simulink model "R_soft_sim2020b"  (R2021a)
settings: Solver=VariableStepAuto  StartTime=0.0  StopTime=10  FixedStep=0.0001  RelTol=1e-3
values from neighbouring files (symbols this model uses):
  beta = 0.1    [computational_time.m]    (also in final_simulation.m; init_script.m)
  beta_r = 0.5    [final_simulation.m]
  D = 0.1    [computational_time.m]    (also in dampingMatrix.m = reshape([0.0,0.0,0.0,0.0,beta,t2,0.0,t2,beta./3.0],[3,3]); final_simulation.m; init_script.m; multiple_frame_plot.m)
  g = 9.81    [computational_time.m]    (also in final_simulation.m; init_script.m)
  k = 1    [computational_time.m]    (also in final_simulation.m; init_script.m = 0.1)
  Kd = -K(2)    [final_simulation.m]
  Kp = -K(1)    [final_simulation.m]
  L = 1    [computational_time.m]    (also in coriolisMatrix.m = ct{1}; final_simulation.m; init_script.m; multiple_frame_plot.m)
  m = 1    [computational_time.m]    (also in coriolisMatrix.m = ct{2}; final_simulation.m; init_script.m)
  theta_dot_init = zeros(3, 1)    [final_simulation.m]
  theta_init = [0; pi/4; -pi/4]    [final_simulation.m]
undefined symbols (not defined in the file or in its folder): alpha_des, collocatedFL, collocatedFL2, DiscIntNeverNeededParam, RSoft_dynamics, Soft_dynamics, thetaR_des
libraries: spsTriangleGeneratorLib x1
settings Model: Creator=Utente  LastModifiedBy=Utente

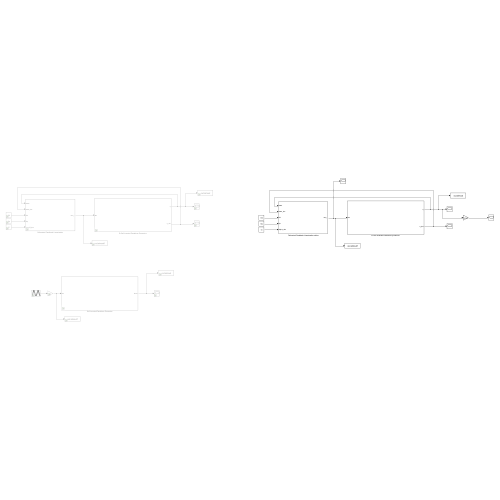
[thumbnail: Simulink's stored preview of the top-level diagram]
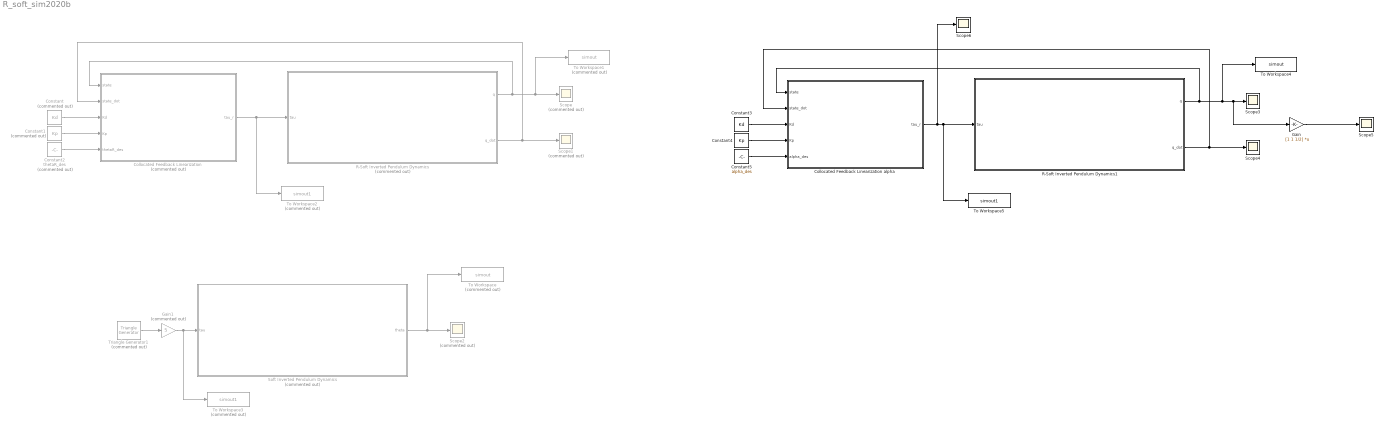
== system R_soft_sim2020b ==
  Collocated Feedback Linearization : Subsystem  Commented=on
  Collocated Feedback Linearization alpha : Subsystem
  Constant : Constant  Commented=on  Value=Kd
  Constant1 : Constant  Commented=on  Value=Kp
  Constant2 : Constant  Commented=on  Value=thetaR_des
  Constant3 : Constant  Value=Kd
  Constant4 : Constant  Value=Kp
  Constant5 : Constant  Value=alpha_des
  Gain : Gain  Gain=[1 1 1/2]  Multiplication=Matrix(K*u) (u vector)
  Gain1 : Gain  Commented=on  Gain=5
  R-Soft Inverted Pendulum Dynamics : Subsystem  Commented=on
  R-Soft Inverted Pendulum Dynamics1 : Subsystem
  Scope : Scope  Commented=on
  Scope1 : Scope  Commented=on
  Scope2 : Scope  Commented=on
  Scope{3..6} (4 alike) : Scope
  Soft Inverted Pendulum Dynamics : Subsystem  Commented=on
  To Workspace : ToWorkspace  Commented=on  VariableName=simout  SaveFormat=Timeseries  SampleTime=-1
  To Workspace1 : ToWorkspace  Commented=on  VariableName=simout  SaveFormat=Timeseries  SampleTime=-1
  To Workspace2 : ToWorkspace  Commented=on  VariableName=simout1  SaveFormat=Timeseries  SampleTime=-1
  To Workspace3 : ToWorkspace  Commented=on  VariableName=simout1  SaveFormat=Timeseries  SampleTime=-1
  To Workspace4 : ToWorkspace  VariableName=simout  SaveFormat=Timeseries  SampleTime=-1
  To Workspace5 : ToWorkspace  VariableName=simout1  SaveFormat=Timeseries  SampleTime=-1
  Triangle Generator1 : spsTriangleGeneratorLib/Triangle Generator  Commented=on  Freq=1/180  Phase=0  Ts=0
  wires:
  Gain1/1 -> To Workspace3/1, Soft Inverted Pendulum Dynamics/1(tau)
  Soft Inverted Pendulum Dynamics/1(theta) -> To Workspace/1, Scope2/1
  Triangle Generator1/1 -> Gain1/1
  R-Soft Inverted Pendulum Dynamics/1(q) -> Collocated Feedback Linearization/1(state), To Workspace1/1, Scope/1
  R-Soft Inverted Pendulum Dynamics/2(q_dot) -> Collocated Feedback Linearization/2(state_dot), Scope1/1
  Collocated Feedback Linearization/1(tau_r) -> To Workspace2/1, R-Soft Inverted Pendulum Dynamics/1(tau)
  Constant/1 -> Collocated Feedback Linearization/3(Kd)
  Constant1/1 -> Collocated Feedback Linearization/4(Kp)
  Constant2/1 -> Collocated Feedback Linearization/5(thetaR_des)
  Collocated Feedback Linearization alpha/1(tau_r) -> Scope6/1, To Workspace5/1, R-Soft Inverted Pendulum Dynamics1/1(tau)
  Constant3/1 -> Collocated Feedback Linearization alpha/3(Kd)
  R-Soft Inverted Pendulum Dynamics1/2(q_dot) -> Collocated Feedback Linearization alpha/2(state_dot), Scope4/1
  Constant4/1 -> Collocated Feedback Linearization alpha/4(Kp)
  Constant5/1 -> Collocated Feedback Linearization alpha/5(alpha_des)
  R-Soft Inverted Pendulum Dynamics1/1(q) -> Collocated Feedback Linearization alpha/1(state), To Workspace4/1, Gain/1, Scope3/1
  Gain/1 -> Scope5/1

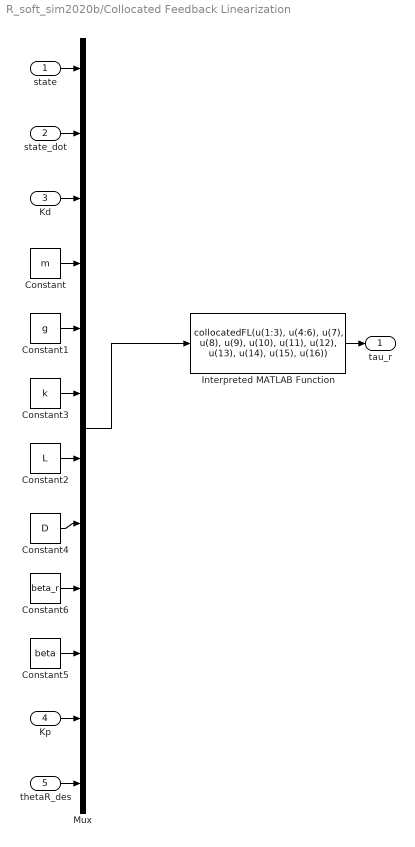
== system R_soft_sim2020b/Collocated Feedback Linearization ==
  state : Inport
  state_dot : Inport  Port=2
  Kd : Inport  Port=3
  Kp : Inport  Port=4
  thetaR_des : Inport  Port=5
  Constant : Constant  Value=m
  Constant1 : Constant  Value=g
  Constant2 : Constant  Value=L
  Constant3 : Constant  Value=k
  Constant4 : Constant  Value=D
  Constant5 : Constant  Value=beta
  Constant6 : Constant  Value=beta_r
  Interpreted MATLAB Function : MATLABFcn  MATLABFcn=collocatedFL(u(1:3), u(4:6), u(7), u(8), u(9), u(10), u(11), u(12), u(13), u(14), u(15), u(16))
  Mux : Mux  Inputs=12
  tau_r : Outport
  wires:
  Mux/1 -> Interpreted MATLAB Function/1
  Kd/1 -> Mux/3
  Constant2/1 -> Mux/7
  Constant1/1 -> Mux/5
  Constant/1 -> Mux/4
  Constant3/1 -> Mux/6
  Interpreted MATLAB Function/1 -> tau_r/1
  state_dot/1 -> Mux/2
  Constant4/1 -> Mux/8
  state/1 -> Mux/1
  thetaR_des/1 -> Mux/12
  Kp/1 -> Mux/11
  Constant5/1 -> Mux/10
  Constant6/1 -> Mux/9

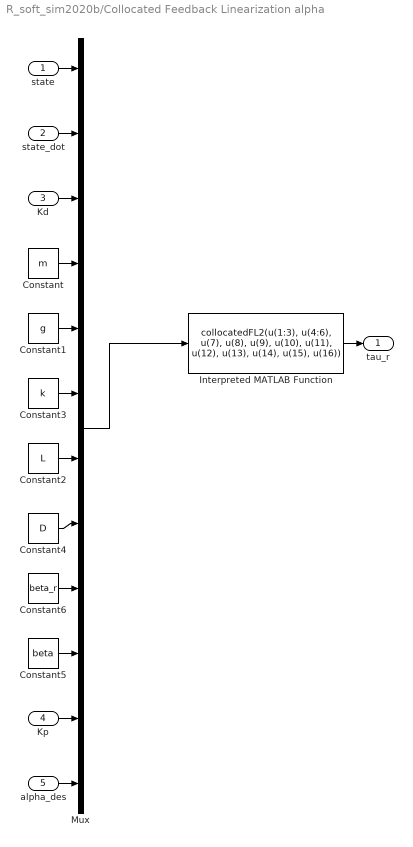
== system R_soft_sim2020b/Collocated Feedback Linearization alpha ==
  state : Inport
  state_dot : Inport  Port=2
  Kd : Inport  Port=3
  Kp : Inport  Port=4
  alpha_des : Inport  Port=5
  Constant : Constant  Value=m
  Constant1 : Constant  Value=g
  Constant2 : Constant  Value=L
  Constant3 : Constant  Value=k
  Constant4 : Constant  Value=D
  Constant5 : Constant  Value=beta
  Constant6 : Constant  Value=beta_r
  Interpreted MATLAB Function : MATLABFcn  MATLABFcn=collocatedFL2(u(1:3), u(4:6), u(7), u(8), u(9), u(10), u(11), u(12), u(13), u(14), u(15), u(16))
  Mux : Mux  Inputs=12
  tau_r : Outport
  wires:
  Mux/1 -> Interpreted MATLAB Function/1
  Kd/1 -> Mux/3
  Constant2/1 -> Mux/7
  Constant1/1 -> Mux/5
  Constant/1 -> Mux/4
  Constant3/1 -> Mux/6
  Interpreted MATLAB Function/1 -> tau_r/1
  state_dot/1 -> Mux/2
  Constant4/1 -> Mux/8
  state/1 -> Mux/1
  alpha_des/1 -> Mux/12
  Kp/1 -> Mux/11
  Constant5/1 -> Mux/10
  Constant6/1 -> Mux/9

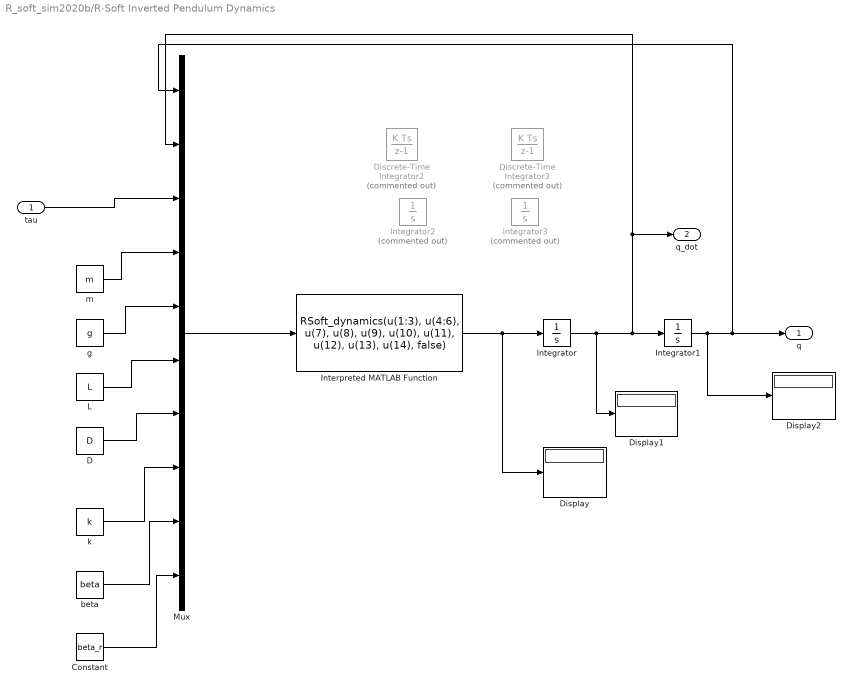
== system R_soft_sim2020b/R-Soft Inverted Pendulum Dynamics ==
  tau : Inport
  Constant : Constant  Value=beta_r
  D : Constant  Value=D
  Discrete-Time Integrator2 : DiscreteIntegrator  Commented=on  InitialCondition=theta_dot_init  SampleTime=-1  ICPrevOutput=DiscIntNeverNeededParam  ICPrevScaledInput=DiscIntNeverNeededParam
  Discrete-Time Integrator3 : DiscreteIntegrator  Commented=on  InitialCondition=theta_init  SampleTime=-1  ICPrevOutput=DiscIntNeverNeededParam  ICPrevScaledInput=DiscIntNeverNeededParam
  Display : Display
  Display1 : Display
  Display2 : Display
  Integrator : Integrator  InitialCondition=theta_dot_init
  Integrator1 : Integrator  InitialCondition=theta_init
  Integrator2 : Integrator  Commented=on  InitialCondition=theta_dot_init
  Integrator3 : Integrator  Commented=on  InitialCondition=theta_init
  Interpreted MATLAB Function : MATLABFcn  MATLABFcn=RSoft_dynamics(u(1:3), u(4:6), u(7), u(8), u(9), u(10), u(11), u(12), u(13), u(14), false)
  L : Constant  Value=L
  Mux : Mux  Inputs=10
  beta : Constant  Value=beta
  g : Constant  Value=g
  k : Constant  Value=k
  m : Constant  Value=m
  q : Outport
  q_dot : Outport  Port=2
  wires:
  Integrator1/1 -> Display2/1, q/1, Mux/1
  g/1 -> Mux/5
  beta/1 -> Mux/9
  k/1 -> Mux/8
  m/1 -> Mux/4
  tau/1 -> Mux/3
  Integrator/1 -> Display1/1, Integrator1/1, q_dot/1, Mux/2
  L/1 -> Mux/6
  D/1 -> Mux/7
  Mux/1 -> Interpreted MATLAB Function/1
  Interpreted MATLAB Function/1 -> Integrator/1, Display/1
  Constant/1 -> Mux/10

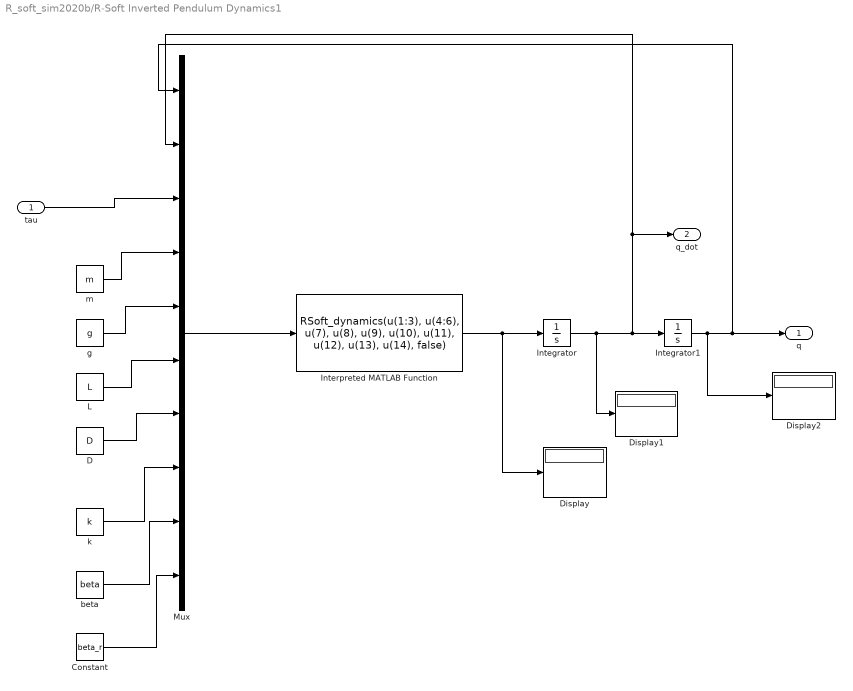
== system R_soft_sim2020b/R-Soft Inverted Pendulum Dynamics1 ==
  tau : Inport
  Constant : Constant  Value=beta_r
  D : Constant  Value=D
  Display : Display
  Display1 : Display
  Display2 : Display
  Integrator : Integrator  InitialCondition=theta_dot_init
  Integrator1 : Integrator  InitialCondition=theta_init
  Interpreted MATLAB Function : MATLABFcn  MATLABFcn=RSoft_dynamics(u(1:3), u(4:6), u(7), u(8), u(9), u(10), u(11), u(12), u(13), u(14), false)
  L : Constant  Value=L
  Mux : Mux  Inputs=10
  beta : Constant  Value=beta
  g : Constant  Value=g
  k : Constant  Value=k
  m : Constant  Value=m
  q : Outport
  q_dot : Outport  Port=2
  wires:
  Integrator1/1 -> Display2/1, q/1, Mux/1
  g/1 -> Mux/5
  beta/1 -> Mux/9
  k/1 -> Mux/8
  m/1 -> Mux/4
  tau/1 -> Mux/3
  Integrator/1 -> Display1/1, Integrator1/1, q_dot/1, Mux/2
  L/1 -> Mux/6
  D/1 -> Mux/7
  Mux/1 -> Interpreted MATLAB Function/1
  Interpreted MATLAB Function/1 -> Integrator/1, Display/1
  Constant/1 -> Mux/10

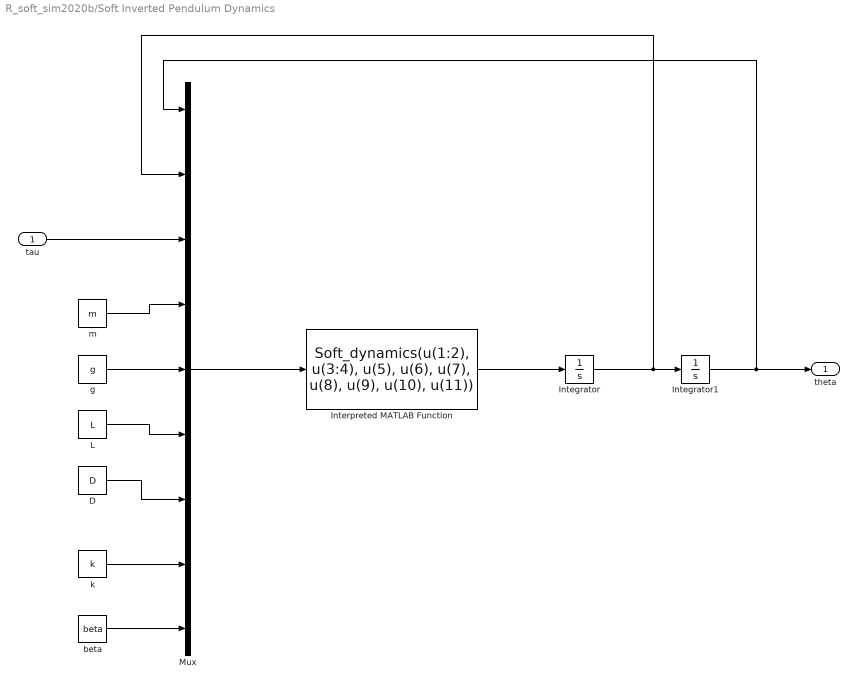
== system R_soft_sim2020b/Soft Inverted Pendulum Dynamics ==
  tau : Inport
  D : Constant  Value=D
  Integrator : Integrator  InitialCondition=theta_dot_init(2:end)
  Integrator1 : Integrator  InitialCondition=theta_init(2:end)
  Interpreted MATLAB Function : MATLABFcn  MATLABFcn=Soft_dynamics(u(1:2), u(3:4), u(5), u(6), u(7), u(8), u(9), u(10), u(11))
  L : Constant  Value=L
  Mux : Mux  Inputs=9
  beta : Constant  Value=beta
  g : Constant  Value=g
  k : Constant  Value=k
  m : Constant  Value=m
  theta : Outport
  wires:
  Integrator1/1 -> theta/1, Mux/1
  g/1 -> Mux/5
  beta/1 -> Mux/9
  k/1 -> Mux/8
  m/1 -> Mux/4
  tau/1 -> Mux/3
  Integrator/1 -> Mux/2, Integrator1/1
  L/1 -> Mux/6
  D/1 -> Mux/7
  Mux/1 -> Interpreted MATLAB Function/1
  Interpreted MATLAB Function/1 -> Integrator/1
